simulink model "impedance_control_test3"  (R2019b)
settings: Solver=VariableStepAuto  StartTime=0.0  StopTime=1  RelTol=1e-3
values from neighbouring files (symbols this model uses):
  a1 = 1    [Dynamics_of_the_System.m]    (also in test_PD.m; test_PD_entrance.m; test_impedence.m)
  a2 = 1    [Dynamics_of_the_System.m]    (also in test_PD.m; test_PD_entrance.m; test_impedence.m)
  friction = 1    [test_PD.m]    (also in test_PD_entrance.m; test_impedence.m)
  IL1 = 1    [equationsofmotion1.m]    (also in test_PD.m; test_PD_entrance.m; test_impedence.m)
  IL2 = 2    [equationsofmotion1.m]    (also in test_PD.m = 1; test_PD_entrance.m = 1; test_impedence.m = 1)
  Im1 = 0.02    [Dynamics_of_the_System.m]    (also in equationsofmotion1.m = 1; test_PD.m = 1; test_PD_entrance.m = 1; test_impedence.m = 1)
  Im2 = 0.02    [Dynamics_of_the_System.m]    (also in equationsofmotion1.m = 2; test_PD.m = 1; test_PD_entrance.m = 1; test_impedence.m = 1)
  K_D = 10    [test_PD.m]    (also in test_PD_entrance.m; test_impedence.m)
  K_P = 10    [test_PD.m]    (also in test_PD_entrance.m; test_impedence.m)
  kr1 = 110    [Dynamics_of_the_System.m]    (also in equationsofmotion1.m = 1; test_PD.m = 1; test_PD_entrance.m = 1; test_impedence.m = 1)
  kr2 = 110    [Dynamics_of_the_System.m]    (also in equationsofmotion1.m = 2; test_PD.m = 1; test_PD_entrance.m = 1; test_impedence.m = 1)
  L1 = 1    [test_PD.m]    (also in test_PD_entrance.m; test_impedence.m)
  L2 = 1    [test_PD.m]    (also in test_PD_entrance.m; test_impedence.m)
  mdx = 1    [test_impedence.m]
  mdy = 1    [test_impedence.m]
  mL1 = 1    [test_PD.m]    (also in test_PD_entrance.m; test_impedence.m)
  mL2 = 1    [test_PD.m]    (also in test_PD_entrance.m; test_impedence.m)
  mm2 = 2    [equationsofmotion1.m]    (also in test_PD.m = 1; test_PD_entrance.m = 1; test_impedence.m = 1)
  qi = [q1 q2]    [PD_entrance.m]    (also in impedance_entrance.m; test_PD.m = [0.5;0.5]; test_PD_entrance.m = [0.5;0.5]; test_impedence.m = [0.5;0.5])
  stiffness = 100    [test_impedence.m]
  xd = [xd1 xd2]    [PD_entrance.m]    (also in impedance_entrance.m; test_PD.m = [1;0]; test_PD_entrance.m = [1;0]; test_impedence.m = [1;0])
  xd_dot = [1;0]    [test_impedence.m]
  xd_doubledot = [1;0]    [test_impedence.m]
  xr = [1;0]    [test_impedence.m]
settings Model: Creator=Danny  LastModifiedBy=Danny

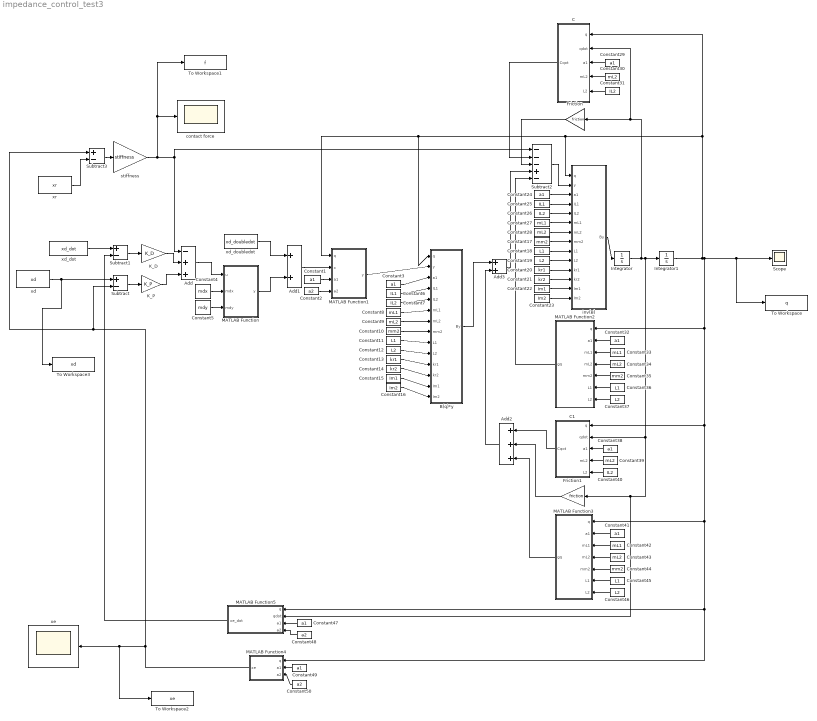
== system impedance_control_test3 ==
  Add : Sum  Inputs=-++
  Add1 : Sum
  Add2 : Sum  Inputs=+++
  Add3 : Sum
  B(q)*y : MATLAB Function  TreatAsAtomicUnit=on
  C : MATLAB Function  TreatAsAtomicUnit=on
  C1 : MATLAB Function  TreatAsAtomicUnit=on
  Constant{1,3,24,29,32,38,41,47,49} (9 alike) : Constant  Value=a1
  Constant{10,17,35,44} (4 alike) : Constant  Value=mm2
  Constant{11,18,36,45} (4 alike) : Constant  Value=L1
  Constant{12,19,37,46} (4 alike) : Constant  Value=L2
  Constant13 : Constant  Value=kr1
  Constant14 : Constant  Value=kr2
  Constant15 : Constant  Value=Im1
  Constant16 : Constant  Value=Im2
  Constant2 : Constant  Value=a2
  Constant20 : Constant  Value=kr1
  Constant21 : Constant  Value=kr2
  Constant22 : Constant  Value=Im1
  Constant23 : Constant  Value=Im2
  Constant25 : Constant  Value=IL1
  Constant{7,26,31,40} (4 alike) : Constant  Value=IL2
  Constant{8,27,33,42} (4 alike) : Constant  Value=mL1
  Constant{9,28,30,34,39,43} (6 alike) : Constant  Value=mL2
  Constant4 : Constant  Value=mdx
  Constant48 : Constant  Value=a2
  Constant5 : Constant  Value=mdy
  Constant50 : Constant  Value=a2
  Constant6 : Constant  Value=IL1
  Friction : Gain  Gain=friction
  Friction1 : Gain  Gain=friction
  Integrator : Integrator  InitialCondition=[0; 0]
  Integrator1 : Integrator  InitialCondition=qi
  K_D : Gain  Gain=K_D
  K_P : Gain  Gain=K_P
  MATLAB Function : MATLAB Function  TreatAsAtomicUnit=on
  MATLAB Function1 : MATLAB Function  TreatAsAtomicUnit=on
  MATLAB Function2 : MATLAB Function  TreatAsAtomicUnit=on
  MATLAB Function3 : MATLAB Function  TreatAsAtomicUnit=on
  MATLAB Function4 : MATLAB Function  TreatAsAtomicUnit=on
  MATLAB Function5 : MATLAB Function  TreatAsAtomicUnit=on
  Scope : Scope
  Subtract : Sum  Inputs=+-
  Subtract1 : Sum  Inputs=+-
  Subtract2 : Sum  Inputs=---+-
  Subtract3 : Sum  Inputs=+-
  To Workspace : ToWorkspace  VariableName=q  SampleTime=-1
  To Workspace1 : ToWorkspace  VariableName=f  SampleTime=-1
  To Workspace2 : ToWorkspace  VariableName=xe  SampleTime=-1
  To Workspace3 : ToWorkspace  VariableName=xd  SampleTime=-1
  contact force : Scope
  inv(B) : MATLAB Function  TreatAsAtomicUnit=on
  stiffness : Gain  Gain=stiffness
  xd : Constant  Value=xd
  xd_dot : Constant  Value=xd_dot
  xd_doubledot : Constant  Value=xd_doubledot
  xe : Scope
  xr : Constant  Value=xr
  wires:
  xd/1 -> To Workspace3/1, Subtract/1
  Constant5/1 -> MATLAB Function/3(mdy)
  MATLAB Function/1(y) -> Add1/2
  K_P/1 -> Add/3
  K_D/1 -> Add/2
  xd_dot/1 -> Subtract1/1
  Subtract/1 -> K_P/1
  Add/1 -> MATLAB Function/1(u)
  xd_doubledot/1 -> Add1/1
  Constant4/1 -> MATLAB Function/2(mdx)
  Subtract1/1 -> K_D/1
  stiffness/1 -> To Workspace1/1, contact force/1, Add/1, Subtract2/1
  Add1/1 -> MATLAB Function1/2(x)
  MATLAB Function1/1(y) -> B(q)*y/2(y)
  inv(B)/1(By) -> Integrator/1
  Integrator/1 -> MATLAB Function5/2(qdot), Friction1/1, C1/2(qdot), Integrator1/1, C/2(qdot), Friction/1
  Subtract2/1 -> inv(B)/2(y)
  Friction/1 -> Subtract2/3
  C/1(Cqot) -> Subtract2/2
  MATLAB Function2/1(gq) -> Subtract2/5
  Integrator1/1 -> MATLAB Function5/1(q), MATLAB Function4/1(q), MATLAB Function3/1(q), C1/1(q), MATLAB Function2/1(q), To Workspace/1, Scope/1, C/1(q), inv(B)/1(q), B(q)*y/1(q), MATLAB Function1/1(q)
  C1/1(Cqot) -> Add2/1
  Friction1/1 -> Add2/2
  MATLAB Function3/1(gq) -> Add2/3
  Add3/1 -> Subtract2/4
  B(q)*y/1(By) -> Add3/1
  Add2/1 -> Add3/2
  MATLAB Function4/1(xe) -> Subtract/2, Subtract3/1, To Workspace2/1, xe/1
  MATLAB Function5/1(xe_dot) -> Subtract1/2
  xr/1 -> Subtract3/2
  Subtract3/1 -> stiffness/1
  Constant1/1 -> MATLAB Function1/3(a1)
  Constant2/1 -> MATLAB Function1/4(a2)
  Constant3/1 -> B(q)*y/3(a1)
  Constant6/1 -> B(q)*y/4(IL1)
  Constant7/1 -> B(q)*y/5(IL2)
  Constant8/1 -> B(q)*y/6(mL1)
  Constant9/1 -> B(q)*y/7(mL2)
  Constant10/1 -> B(q)*y/8(mm2)
  Constant11/1 -> B(q)*y/9(L1)
  Constant12/1 -> B(q)*y/10(L2)
  Constant13/1 -> B(q)*y/11(kr1)
  Constant15/1 -> B(q)*y/13(Im1)
  Constant14/1 -> B(q)*y/12(kr2)
  Constant16/1 -> B(q)*y/14(Im2)
  Constant24/1 -> inv(B)/3(a1)
  Constant25/1 -> inv(B)/4(IL1)
  Constant26/1 -> inv(B)/5(IL2)
  Constant27/1 -> inv(B)/6(mL1)
  Constant28/1 -> inv(B)/7(mL2)
  Constant17/1 -> inv(B)/8(mm2)
  Constant18/1 -> inv(B)/9(L1)
  Constant19/1 -> inv(B)/10(L2)
  Constant20/1 -> inv(B)/11(kr1)
  Constant21/1 -> inv(B)/12(kr2)
  Constant22/1 -> inv(B)/13(Im1)
  Constant23/1 -> inv(B)/14(Im2)
  Constant29/1 -> C/3(a1)
  Constant30/1 -> C/4(mL2)
  Constant31/1 -> C/5(L2)
  Constant32/1 -> MATLAB Function2/2(a1)
  Constant33/1 -> MATLAB Function2/3(mL1)
  Constant34/1 -> MATLAB Function2/4(mL2)
  Constant35/1 -> MATLAB Function2/5(mm2)
  Constant36/1 -> MATLAB Function2/6(L1)
  Constant37/1 -> MATLAB Function2/7(L2)
  Constant38/1 -> C1/3(a1)
  Constant39/1 -> C1/4(mL2)
  Constant40/1 -> C1/5(L2)
  Constant41/1 -> MATLAB Function3/2(a1)
  Constant46/1 -> MATLAB Function3/7(L2)
  Constant45/1 -> MATLAB Function3/6(L1)
  Constant43/1 -> MATLAB Function3/4(mL2)
  Constant42/1 -> MATLAB Function3/3(mL1)
  Constant44/1 -> MATLAB Function3/5(mm2)
  Constant47/1 -> MATLAB Function5/3(a1)
  Constant48/1 -> MATLAB Function5/4(a2)
  Constant49/1 -> MATLAB Function4/2(a1)
  Constant50/1 -> MATLAB Function4/3(a2)

== matlab function impedance_control_test3/MATLAB Function1 ==
  data: q input; y output; x input; a1 input; a2 input
function y = fcn(q,x,a1,a2)
Ja = [-a1*sin(q(1))-a2*sin(q(1)+q(2)), -a2*sin(q(1)+q(2));
    a1*cos(q(1))+a2*cos(q(1)+q(2)), a2*cos(q(1)+q(2))];
y = inv(Ja)*x;

== matlab function impedance_control_test3/MATLAB Function ==
  data: u input; y output; mdx input; mdy input
function y = fcn(u,mdx,mdy)
Md = [mdx 0; 0 mdy];
y = u'*inv(Md);

== matlab function impedance_control_test3/B(q)*y ==
  data: q input; By output; y input; a1 input; IL1 input; IL2 input; mL1 input; mL2 input; mm2 input; L1 input; L2 input; kr1 input; kr2 input; Im1 input; Im2 input
function By = fcn(q,y,a1, IL1, IL2, mL1, mL2 ,mm2, L1, L2, kr1, kr2, Im1, Im2)
b11 = IL1 + mL1*(L1.^2) + (kr1.^2)*Im1 + IL2 +... 
    mL2*(a1.^2 + L2.^2 + 2*a1*L2*cos(q(2))) + Im2 +mm2*(a1.^2);
b12 = IL2 + mL2*(L2.^2 + a1*L2*cos(q(2))) + kr2*Im2;
b21 = b12;
b22 = IL2 + mL2*L2.^2 + (kr2.^2)*Im2;
B = [b11 b12; b21 b22];
By = B*y;

== matlab function impedance_control_test3/inv(B) ==
  data: q input; By output; y input; a1 input; IL1 input; IL2 input; mL1 input; mL2 input; mm2 input; L1 input; L2 input; kr1 input; kr2 input; Im1 input; Im2 input
function By = fcn(q,y,a1,IL1,IL2,mL1,mL2,mm2,L1,L2,kr1,kr2,Im1,Im2)
if nargin==1
    q = [0.5*pi;0.5*pi];
end

b11 = IL1 + mL1*(L1.^2) + (kr1.^2)*Im1 + IL2 +... 
    mL2*(a1.^2 + L2.^2 + 2*a1*L2*cos(q(2))) + Im2 +mm2*(a1.^2);
b12 = IL2 + mL2*(L2.^2 + a1*L2*cos(q(2))) + kr2*Im2;
b21 = b12;
b22 = IL2 + mL2*L2.^2 + (kr2.^2)*Im2;
B = [b11 b12; b21 b22];
By = inv(B)*y;

== matlab function impedance_control_test3/C ==
  data: q input; Cqot output; qdot input; a1 input; mL2 input; L2 input
function Cqot = fcn(q,qdot,a1,mL2,L2)
c11 = (-mL2*a1*L2*sin(q(2)))*qdot(2);
c12 = (-mL2*a1*L2*sin(q(2)))*(qdot(1)+qdot(2));
c21 = -(-mL2*a1*L2*sin(q(2)))*qdot(1);
c22 = 0;
C = [c11 c12; c21 c22];
Cqot = C*qdot;

== matlab function impedance_control_test3/MATLAB Function2 ==
  data: q input; gq output; a1 input; mL1 input; mL2 input; mm2 input; L1 input; L2 input
function gq = fcn(q,a1,mL1,mL2,mm2,L1,L2)
g = 9.81;
g1 = (mL1*L1 + mm2*a1 + mL2*a1)*g*cos(q(1)) + mL2*L2*g*cos(q(1)+q(2));
g2 = mL2*L2*g*cos(q(1)+q(2));
gq = [g1;g2];

== matlab function impedance_control_test3/C1 ==
  data: q input; Cqot output; qdot input; a1 input; mL2 input; L2 input
function Cqot = fcn(q,qdot,a1,mL2,L2)
c11 = (-mL2*a1*L2*sin(q(2)))*qdot(2);
c12 = (-mL2*a1*L2*sin(q(2)))*(qdot(1)+qdot(2));
c21 = -(-mL2*a1*L2*sin(q(2)))*qdot(1);
c22 = 0;
C = [c11 c12; c21 c22];
Cqot = C*qdot;

== matlab function impedance_control_test3/MATLAB Function3 ==
  data: q input; gq output; a1 input; mL1 input; mL2 input; mm2 input; L1 input; L2 input
function gq = fcn(q,a1,mL1,mL2,mm2,L1,L2)
g = 9.81;
g1 = (mL1*L1 + mm2*a1 + mL2*a1)*g*cos(q(1)) + mL2*L2*g*cos(q(1)+q(2));
g2 = mL2*L2*g*cos(q(1)+q(2));
gq = [g1;g2];

== matlab function impedance_control_test3/MATLAB Function5 ==
  data: q input; xe_dot output; qdot input; a1 input; a2 input
function xe_dot = fcn(q,qdot,a1,a2)
Ja = [-a1*sin(q(1))-a2*sin(q(1)+q(2)), -a2*sin(q(1)+q(2));
       a1*cos(q(1))+a2*cos(q(1)+q(2)), a2*cos(q(1)+q(2))];
xe_dot = Ja*qdot;

== matlab function impedance_control_test3/MATLAB Function4 ==
  data: q input; xe output; a1 input; a2 input
function xe = fcn(q,a1,a2)
xe = [a1*cos(q(1))+a2*cos(q(1)+q(2));
    a1*sin(q(1))+a2*sin(q(1)+q(2))];
